simulink model "Bio_fed_batch"  (R2020b)
settings: Solver=daessc  StartTime=0.0  StopTime=50  FixedStep=0.01  MaxStep=0.1  MinStep=0.01  RelTol=1e-3
undefined symbols (not defined in the file or in its folder): sigbuilder_block
libraries: pid_lib x1
settings Model: Creator=César-Garech  LastModifiedBy=César-Garech

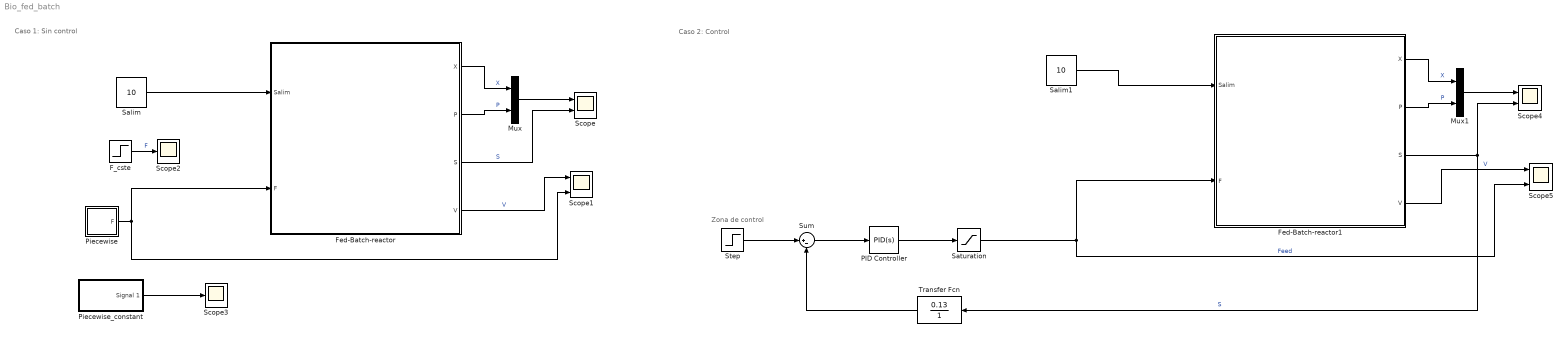
== system Bio_fed_batch ==
  note: Caso 2: Control
  note: Zona de control
  note: Caso 1: Sin control
  F_cste : Step  Time=20  After=0.1  SampleTime=0
  Fed-Batch-reactor : Subsystem
      mask Display: image('biorreactor.png'); % Use "Edit Image" on toolstrip to change.
  Fed-Batch-reactor1 : Subsystem
      mask Display: image('biorreactor.png'); % Use "Edit Image" on toolstrip to change.
  Mux : Mux  Inputs=2
  Mux1 : Mux  Inputs=2
  PID Controller : pid_lib/PID Controller  Controller=PID  Form=Parallel  TimeDomain=Continuous-time  UseExternalTs=off  SampleTime=-1  IntegratorMethod=Forward Euler  FilterMethod=Forward Euler  ControllerParametersSource=internal  P=0.228837975645856  I=0.0141490916683521  D=0.340888422114362  UseFilter=on  N=0.458051925527811  TunerSelectOption=Transfer Function Based (PID Tuner App)  InitialConditionSource=internal  InitialConditionForIntegrator=0  InitialConditionForFilter=0  DifferentiatorICPrevScaledInput=0  ExternalReset=none  TrackingMode=off  Kt=1  LimitOutput=off  SatLimitsSource=internal  UpperSaturationLimit=inf  LowerSaturationLimit=-inf  LinearizeAsGain=on  AntiWindupMode=none  Kb=1  POutMin=[]  POutMax=[]  IOutMin=[]  IOutMax=[]  DOutMin=[]  DOutMax=[]  NOutMin=[]  NOutMax=[]  SumOutMin=[]  SumOutMax=[]  SaturationOutMin=[]  SaturationOutMax=[]  PParamMin=[]  PParamMax=[]  IParamMin=[]  IParamMax=[]  DParamMin=[]  DParamMax=[]  NParamMin=[]  NParamMax=[]  KbParamMin=[]  KbParamMax=[]  KtParamMin=[]  KtParamMax=[]  KbOutMin=[]  KbOutMax=[]  KtOutMin=[]  KtOutMax=[]  IntegratorOutMin=[]  IntegratorOutMax=[]  FilterOutMin=[]  FilterOutMax=[]  SumI1OutMin=[]  SumI1OutMax=[]  SumI2OutMin=[]  SumI2OutMax=[]  SumI3OutMin=[]  SumI3OutMax=[]  SumI4OutMin=[]  SumI4OutMax=[]  SumDOutMin=[]  SumDOutMax=[]  DifferentiatorOutMin=[]  DifferentiatorOutMax=[]  FilterDiffOutCoefMin=[]  FilterDiffOutCoefMax=[]  ReciprocalOutMin=[]  ReciprocalOutMax=[]  SumDenOutMin=[]  SumDenOutMax=[]  SumNumOutMin=[]  SumNumOutMax=[]  DivideOutMin=[]  DivideOutMax=[]  UdiffTsProdOutMin=[]  UdiffTsProdOutMax=[]  NTsProdOutMin=[]  NTsProdOutMax=[]  UintegralTsProdOutMin=[]  UintegralTsProdOutMax=[]  UngainTsProdOutMin=[]  UngainTsProdOutMax=[]  IntegratorContinuousStateAttributes=''  IntegratorStateMustResolveToSignalObject=off  IntegratorRTWStateStorageClass=Auto  FilterContinuousStateAttributes=''  FilterStateMustResolveToSignalObject=off  FilterRTWStateStorageClass=Auto  ParallelPVariant=InternalParameters  IdealPVariant=Disabled  IVariant=InternalParameters  DVariant=InternalParameters  IntegratorVariant=Continuous  SatVariant=Disabled  AWVariant=Passthrough  PCopyVariant=Disabled  TRVariant=Disabled  FdbkBlocksVariant=Forward  IdealPFdbkVariant=Disabled  SatFdbkVariant=Disabled  DerivativeFilterVariant=ContFilter  NVariant=InternalParameters  NCopyVariant=Disabled  FilterICVariant=InternalICsFilter  IntegratorICVariant=InternalICs  ExternalResetVariant=Disabled  TRSumVariant=Passthrough  SumFdbkVariant=Disabled  SumVariant=Sum_PID  TsampFilterVariant=InternalTs  TsampNgainVariant=Passthrough  TsampIntegralVariant=Passthrough  ExternalSaturationOutDataTypeStr=Inherit: Same as second input
  Piecewise : Subsystem
  Piecewise_constant : Subsystem  Tag=STV Subsys  LoadFcn=sigbuilder_block('load');  StartFcn=sigbuilder_block('start');  StopFcn=sigbuilder_block('stop');  ClipboardFcn=sigbuilder_block('clipboard');  mask(Sigbuilder block){tuvar=[0:10]}
      mask help: Simulink:masks:SigbuilderBlock_MD
      mask init:
      | if ~strcmp(get_param(bdroot(gcbh),'SimulationStatus'),'stopped') tuvar = sigbuilder_block('maskInit'); end
      settings: CopyFcn=sigbuilder_block('copy');  DeleteFcn=sigbuilder_block('delete');  ModelCloseFcn=sigbuilder_block('modelClose');  PreSaveFcn=sigbuilder_block('preSave');  PauseFcn=sigbuilder_block('pause');  ContinueFcn=sigbuilder_block('continue');  NameChangeFcn=sigbuilder_block('namechange');  OpenFcn=sigbuilder_block('open',[423 130.2 550.8 400.2 ]);  CloseFcn=sigbuilder_block('close');
      mask Display: plot(0, 0, 100, 100,[2, 2, 32, 32, 2], [68, 8, 8, 68, 68],[32, 2], [38, 38], [32, 19, 2],[53, 60, 44], [32, 17, 17, 2],[16, 16, 31, 31]);txt = getActiveGroup(gcbh);text(2, 100, txt,'verticalAlignment', 'top');
  Salim : Constant  Value=10  VectorParams1D=off  SampleTime=-1
  Salim1 : Constant  Value=10  VectorParams1D=off  SampleTime=-1
  Saturation : Saturate  UpperLimit=10  LowerLimit=0
  Scope{,1,4..5} (4 alike) : Scope  NumInputPorts=2
  Scope2 : Scope
  Scope3 : Scope
  Step : Step  Time=15  Before=0.01  After=10  SampleTime=0
  Sum : Sum  Inputs=|+-
  Transfer Fcn : TransferFcn  Numerator=[0.13]  Denominator=[1]
  wires:
  Mux/1 -> Scope/1
  Fed-Batch-reactor/1(X) -> Mux/1  "X"
  Fed-Batch-reactor/3(S) -> Scope/2  "S"
  Fed-Batch-reactor/2(P) -> Mux/2  "P"
  Salim/1 -> Fed-Batch-reactor/1(Salim)
  Fed-Batch-reactor/4(V) -> Scope1/1  "V"
  Piecewise/1(F) -> Scope1/2, Fed-Batch-reactor/2(F)
  Piecewise_constant/1(Signal 1) -> Scope3/1
  F_cste/1 -> Scope2/1  "F"
  Fed-Batch-reactor1/3(S) -> Scope4/2, Transfer Fcn/1  "S"
  Fed-Batch-reactor1/4(V) -> Scope5/1  "V"
  Fed-Batch-reactor1/2(P) -> Mux1/2  "P"
  Mux1/1 -> Scope4/1
  Salim1/1 -> Fed-Batch-reactor1/1(Salim)
  Fed-Batch-reactor1/1(X) -> Mux1/1  "X"
  Sum/1 -> PID Controller/1
  Transfer Fcn/1 -> Sum/2
  Saturation/1 -> Fed-Batch-reactor1/2(F), Scope5/2  "Feed"
  PID Controller/1 -> Saturation/1
  Step/1 -> Sum/1

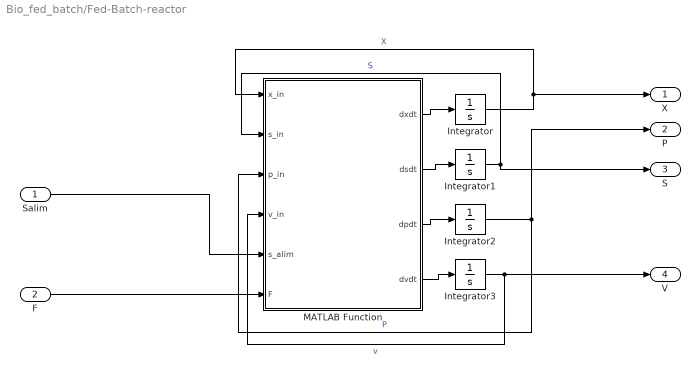
== system Bio_fed_batch/Fed-Batch-reactor ==
  Salim : Inport
  F : Inport  Port=2
  Integrator : Integrator  InitialCondition=0.01
  Integrator1 : Integrator  InitialCondition=20
  Integrator2 : Integrator
  Integrator3 : Integrator  InitialCondition=1
  MATLAB Function : MATLAB Function  TreatAsAtomicUnit=on
  X : Outport
  P : Outport  Port=2
  S : Outport  Port=3
  V : Outport  Port=4
  wires:
  MATLAB Function/3(dpdt) -> Integrator2/1
  Integrator/1 -> X/1, MATLAB Function/1(x_in)  "X"
  Integrator2/1 -> P/1, MATLAB Function/3(p_in)  "P"
  MATLAB Function/2(dsdt) -> Integrator1/1
  MATLAB Function/1(dxdt) -> Integrator/1
  Integrator1/1 -> S/1, MATLAB Function/2(s_in)  "S"
  MATLAB Function/4(dvdt) -> Integrator3/1
  Integrator3/1 -> V/1, MATLAB Function/4(v_in)  "v"
  Salim/1 -> MATLAB Function/5(s_alim)
  F/1 -> MATLAB Function/6(F)

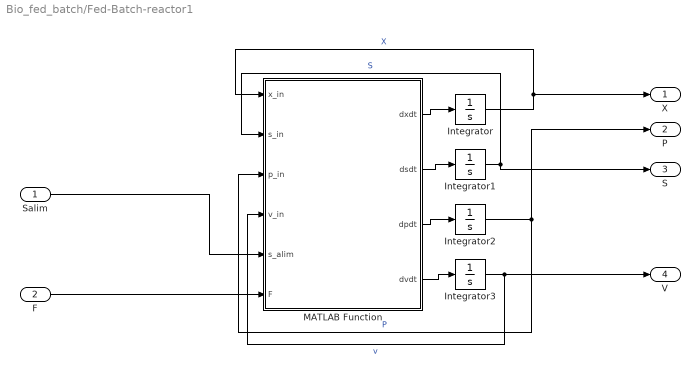
== system Bio_fed_batch/Fed-Batch-reactor1 ==
  Salim : Inport
  F : Inport  Port=2
  Integrator : Integrator  InitialCondition=0.01
  Integrator1 : Integrator  InitialCondition=20
  Integrator2 : Integrator
  Integrator3 : Integrator  InitialCondition=1
  MATLAB Function : MATLAB Function  TreatAsAtomicUnit=on
  X : Outport
  P : Outport  Port=2
  S : Outport  Port=3
  V : Outport  Port=4
  wires:
  MATLAB Function/3(dpdt) -> Integrator2/1
  Integrator/1 -> X/1, MATLAB Function/1(x_in)  "X"
  Integrator2/1 -> P/1, MATLAB Function/3(p_in)  "P"
  MATLAB Function/2(dsdt) -> Integrator1/1
  MATLAB Function/1(dxdt) -> Integrator/1
  Integrator1/1 -> S/1, MATLAB Function/2(s_in)  "S"
  MATLAB Function/4(dvdt) -> Integrator3/1
  Integrator3/1 -> V/1, MATLAB Function/4(v_in)  "v"
  Salim/1 -> MATLAB Function/5(s_alim)
  F/1 -> MATLAB Function/6(F)

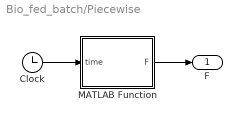
== system Bio_fed_batch/Piecewise ==
  Clock : Clock
  MATLAB Function : MATLAB Function  TreatAsAtomicUnit=on
  F : Outport
  wires:
  Clock/1 -> MATLAB Function/1(time)
  MATLAB Function/1(F) -> F/1

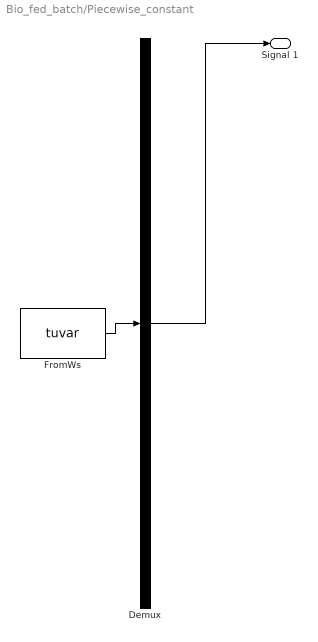
== system Bio_fed_batch/Piecewise_constant ==
  Demux : Demux  Tag=STV Demux  Outputs=1
      settings: DisplayOption=none
  FromWs : FromWorkspace  Tag=STV FromWs  VariableName=tuvar
      SigBuilderData=|
      | common.afterFinalStr = 'Extrapolate'
      | common.sampleTime = 0
      | dataSet.timeRange = [0 32]
      | dataSet.name = 'Group 1'
      | sbobj.Groups.Name = 'Group 1'
      | sbobj.Groups.Signals.Name = 'Signal 1'
      | sbobj.Groups.Signals.XData = [0 10 10 14.95 14.95 32]
      | sbobj.Groups.Signals.YData = [0 0 0.295 0.79 0 0]
      | sbobj.Groups.TimeRange = [0 32]
  Signal 1 : Outport  Tag=STV Outport
  wires:
  Demux/1 -> Signal 1/1
  FromWs/1 -> Demux/1

== matlab function Bio_fed_batch/Piecewise/MATLAB Function ==
  data: time input; F output
function F = Flow(time)



if time<=10
    F=0;
elseif time>10 && time<=15
    F=0.1;
elseif time>15 && time<=20
    F=0.1;
elseif time>20 && time<=30
    F=0.8;
else
    F=0;
end


end

== matlab function Bio_fed_batch/Fed-Batch-reactor/MATLAB Function ==
  data: x_in input; dxdt output; s_in input; p_in input; dsdt output; dpdt output; v_in input; dvdt output; s_alim input; F input
function [dxdt, dsdt,dpdt,dvdt] =Bio_fed_batch(x_in,s_in,p_in,v_in,s_alim,F)

%Definir Parámetros
umax=0.75;%h^-1Velocidad de crecimiento máximo
Ks=0.08; %Afininidad por el sustrato
Smax=30; %Sustrato máximo que inhibie el crecimiento
Yxs=0.8;% (gX/gS) rendimiento de biomasa en sustrato
ms=0.00001; %constante de mantenimiento
alfa=0.05; %constante asociada al crecimiento
beta=0.002; %constante no asociada al crecimiento

%Condiciones iniciales
x=x_in;
s=s_in;
p=p_in;
v=v_in;


%Ecuaciones constitutivas
u=umax*(s/(Ks+s)*(1-(s/Smax))); %h^-1
Rx=u*x;
Rs=(u/(Yxs)+ms)*x;
Rp=(alfa*u+beta)*x;

%Balances
dxdt=Rx-(F/v)*x;
dsdt=-Rs+(F/v)*(s_alim-s);
dpdt=Rp-(F/v)*p;
dvdt=F;

end

== matlab function Bio_fed_batch/Fed-Batch-reactor1/MATLAB Function ==
  data: x_in input; dxdt output; s_in input; p_in input; dsdt output; dpdt output; v_in input; dvdt output; s_alim input; F input
function [dxdt, dsdt,dpdt,dvdt] =Bio_fed_batch(x_in,s_in,p_in,v_in,s_alim,F)

%Definir Parámetros
umax=0.75;%h^-1Velocidad de crecimiento máximo
Ks=0.08; %Afininidad por el sustrato
Smax=30; %Sustrato máximo que inhibie el crecimiento
Yxs=0.8;% (gX/gS) rendimiento de biomasa en sustrato
ms=0.00001; %constante de mantenimiento
alfa=0.05; %constante asociada al crecimiento
beta=0.002; %constante no asociada al crecimiento

%Condiciones iniciales
x=x_in;
s=s_in;
p=p_in;
v=v_in;


%Ecuaciones constitutivas
u=umax*(s/(Ks+s)*(1-(s/Smax))); %h^-1
Rx=u*x;
Rs=(u/(Yxs)+ms)*x;
Rp=(alfa*u+beta)*x;

%Balances
dxdt=Rx-(F/v)*x;
dsdt=-Rs+(F/v)*(s_alim-s);
dpdt=Rp-(F/v)*p;
dvdt=F;

end
